simulink model "PlantSimulationLABC_V3_R2019b"  (R2019b)
settings: Solver=ode4  StartTime=0.0  StopTime=10  FixedStep=1e-4  RelTol=1e-3
undefined symbols (not defined in the file or in its folder): Kd, Ki, Kp, T
libraries: simulink x2
settings Model: EnablePacing=on  Creator=jenei  LastModifiedBy=Marcelo
settings SFSimCC: CustomCodeUndefinedFunction=UseInterfaceOnly

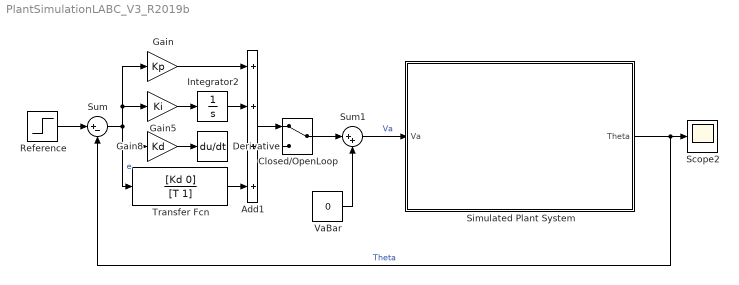
== system PlantSimulationLABC_V3_R2019b ==
  Add1 : Sum  Inputs=++++
  Closed/OpenLoop : ManualSwitch
  Derivative : Derivative
  Gain : Gain  Gain=Kp
  Gain5 : Gain  Gain=Ki
  Gain8 : Gain  Gain=Kd
  Integrator2 : Integrator
  Reference : Step  Time=5  Before=-45  After=-30  SampleTime=0
  Scope2 : Scope
  Simulated Plant System : Subsystem  mask{l=0, m=0, kp=0, b=0, vabar=0}
      mask init:
      | l = 0.15; % [m]
      | m = 0.15; % [kg]
      | Kp = 0.15; % [s*A/m]
      | b = 0.2; % [kg*m/s]
      | syms x
      | vabar = solve((Kp/m)*x^2-9.8*cos(deg2rad(-45)) == 0);
      | vabar = abs(double(vabar(1)));
  Sum : Sum  Inputs=|+-
  Sum1 : Sum  Inputs=|++
  Transfer Fcn : TransferFcn  Numerator=[Kd 0]  Denominator=[T 1]
  VaBar : Constant  Value=0
  wires:
  Simulated Plant System/1(Theta) -> Sum/2, Scope2/1  "Theta"
  VaBar/1 -> Sum1/2
  Closed/OpenLoop/1 -> Sum1/1
  Sum1/1 -> Simulated Plant System/1(Va)  "Va"
  Sum/1 -> Gain5/1, Gain/1, Gain8/1, Transfer Fcn/1  "e"
  Add1/1 -> Closed/OpenLoop/1
  Transfer Fcn/1 -> Add1/4
  Gain5/1 -> Integrator2/1
  Integrator2/1 -> Add1/2
  Gain8/1 -> Derivative/1
  Gain/1 -> Add1/1
  Reference/1 -> Sum/1

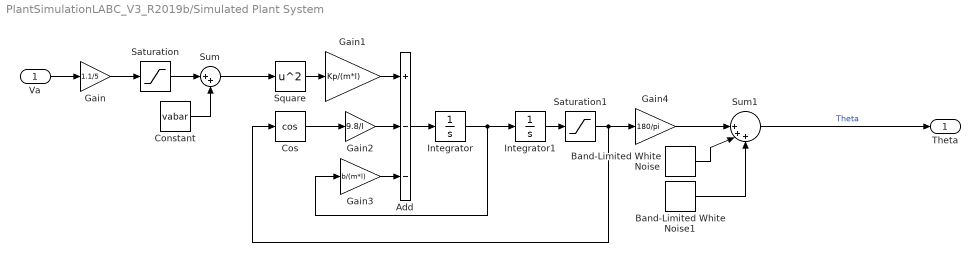
== system PlantSimulationLABC_V3_R2019b/Simulated Plant System ==
  Va : Inport
  Add : Sum  Inputs=+--
  Band-Limited White Noise : simulink/Sources/Band-Limited White Noise  Cov=[0.00005]  Ts=0.05  seed=[23341]
  Band-Limited White Noise1 : simulink/Sources/Band-Limited White Noise  Cov=[0.01]  Ts=1  seed=[23341]
  Constant : Constant  Value=vabar
  Cos : Trigonometry  Operator=cos
  Gain : Gain  Gain=1.1/5
  Gain1 : Gain  Gain=Kp/(m*l)
  Gain2 : Gain  Gain=9.8/l
  Gain3 : Gain  Gain=b/(m*l)
  Gain4 : Gain  Gain=180/pi
  Integrator : Integrator
  Integrator1 : Integrator  InitialCondition=deg2rad(-45)
  Saturation : Saturate  UpperLimit=3  LowerLimit=0
  Saturation1 : Saturate  UpperLimit=deg2rad(90)  LowerLimit=deg2rad(-45)
  Square : Math  Operator=square  SaturateOnIntegerOverflow=on
  Sum : Sum  Inputs=|++
  Sum1 : Sum  Inputs=||+++
  Theta : Outport
  wires:
  Gain4/1 -> Sum1/1
  Integrator/1 -> Integrator1/1, Gain3/1
  Band-Limited White Noise/1 -> Sum1/2
  Add/1 -> Integrator/1
  Gain1/1 -> Add/1
  Integrator1/1 -> Saturation1/1
  Gain2/1 -> Add/2
  Square/1 -> Gain1/1
  Cos/1 -> Gain2/1
  Sum1/1 -> Theta/1  "Theta"
  Gain3/1 -> Add/3
  Band-Limited White Noise1/1 -> Sum1/3
  Constant/1 -> Sum/2
  Gain/1 -> Saturation/1
  Va/1 -> Gain/1
  Saturation1/1 -> Cos/1, Gain4/1
  Sum/1 -> Square/1
  Saturation/1 -> Sum/1
